simulink model "RailP_DD"  (R2018a)
settings: configuration reference "cs_ert" (kept outside this file)
model workspace (MAT data in the model file):
  RailP_DD_DT = 10
values from neighbouring files (symbols this model uses):
  RailP_pLin_CUR : value not decoded    [RailP_DD.sldd]
  RailP_pLin_CURX : value not decoded    [RailP_DD.sldd]
  RailP_tiSRCMaxDefDeb_C = 200.0    [RailP_DD.sldd]
  RailP_tiSRCMaxOKDeb_C = 200.0    [RailP_DD.sldd]
  RailP_tiSRCMinDefDeb_C = 200.0    [RailP_DD.sldd]
  RailP_tiSRCMinOKDeb_C = 200.0    [RailP_DD.sldd]
  RailP_uSRCMax_C = 4700.0    [RailP_DD.sldd]
  RailP_uSRCMin_C = 131.0    [RailP_DD.sldd]
libraries: sllib x2
settings Model: DataDictionary=RailP_DD.sldd  Creator=zhoutinglin  LastModifiedBy=zhoutinglin

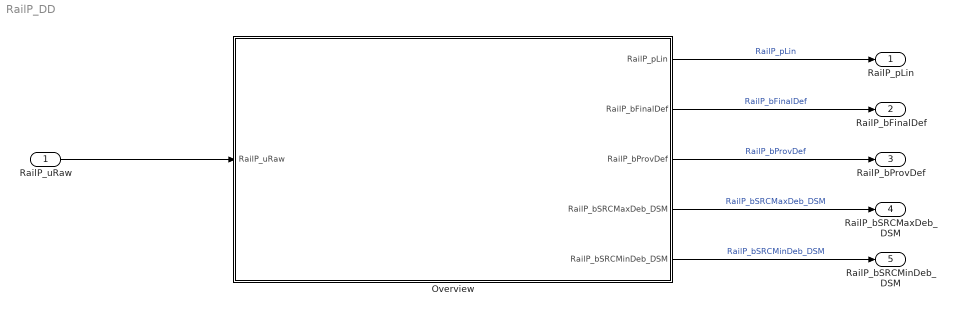
== system RailP_DD ==
  RailP_uRaw : Inport  Description=Status of FId_RailPSS  OutMin=0  OutMax=5000  OutDataTypeStr=Volt_mV  PortDimensions=[1 1]
  Overview : Subsystem
  RailP_pLin : Outport
  RailP_bFinalDef : Outport  Port=2
  RailP_bProvDef : Outport  Port=3
  RailP_bSRCMaxDeb_DSM : Outport  Port=4
  RailP_bSRCMinDeb_DSM : Outport  Port=5
  wires:
  RailP_uRaw/1 -> Overview/1(RailP_uRaw)
  Overview/1(RailP_pLin) -> RailP_pLin/1  "RailP_pLin"
  Overview/2(RailP_bFinalDef) -> RailP_bFinalDef/1  "RailP_bFinalDef"
  Overview/3(RailP_bProvDef) -> RailP_bProvDef/1  "RailP_bProvDef"
  Overview/4(RailP_bSRCMaxDeb_DSM) -> RailP_bSRCMaxDeb_DSM/1  "RailP_bSRCMaxDeb_DSM"
  Overview/5(RailP_bSRCMinDeb_DSM) -> RailP_bSRCMinDeb_DSM/1  "RailP_bSRCMinDeb_DSM"

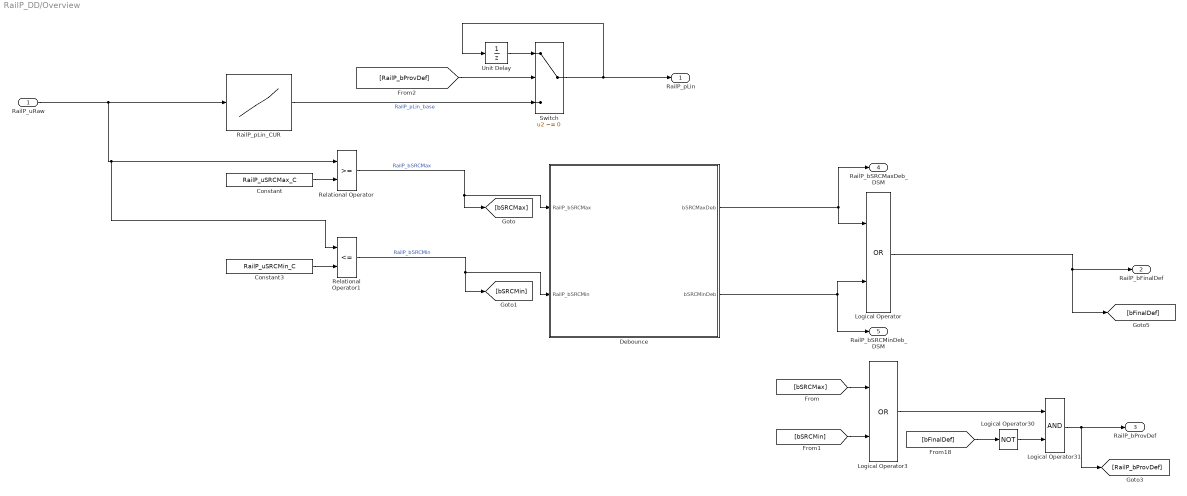
== system RailP_DD/Overview ==
  RailP_uRaw : Inport  Tag=mv
  Constant : Constant  Value=RailP_uSRCMax_C
  Constant3 : Constant  Value=RailP_uSRCMin_C
  Debounce : Subsystem
  Logical Operator : Logic  Operator=OR  AllPortsSameDT=off  OutDataTypeStr=boolean
  Logical Operator3 : Logic  Operator=OR  AllPortsSameDT=off  OutDataTypeStr=boolean
  Logical Operator30 : Logic  Operator=NOT  AllPortsSameDT=off  OutDataTypeStr=boolean
  Logical Operator31 : Logic  AllPortsSameDT=off  OutDataTypeStr=boolean
  RailP_pLin_CUR : Lookup_n-D  NumberOfTableDimensions=1  BreakpointsForDimension1=RailP_pLin_CURX  IndexSearchMethod=Linear search  BeginIndexSearchUsingPreviousIndexResult=on  UseOneInputPortForAllInputData=on  Table=RailP_pLin_CUR  ExtrapMethod=Clip  UseLastTableValue=on  InternalRulePriority=Speed  OutDataTypeStr=Inherit: Inherit via back propagation  SaturateOnIntegerOverflow=on
  Relational Operator : RelationalOperator  OutDataTypeStr=boolean  RndMeth=Nearest  InputSameDT=on
  Relational Operator1 : RelationalOperator  Operator=<=  OutDataTypeStr=boolean  RndMeth=Nearest  InputSameDT=on
  Switch : Switch  Criteria=u2 ~= 0
  Unit Delay : UnitDelay  SampleTime=-1
      settings: AttributesFormatString=InitialValue=%<InitialCondition>
  RailP_pLin : Outport  Tag=bar
  RailP_bFinalDef : Outport  Port=2
  RailP_bProvDef : Outport  Port=3
  RailP_bSRCMaxDeb_DSM : Outport  Port=4
  RailP_bSRCMinDeb_DSM : Outport  Port=5
  wires:
  Relational Operator1/1 -> [bSRCMin], Debounce/2(RailP_bSRCMin)  "RailP_bSRCMin"
  RailP_pLin_CUR/1 -> Switch/3  "RailP_pLin_base"
  [RailP_bProvDef] -> Switch/2
  Constant/1 -> Relational Operator/2
  Debounce/2(bSRCMinDeb) -> Logical Operator/2, RailP_bSRCMinDeb_DSM/1
  Switch/1 -> Unit Delay/1, RailP_pLin/1
  Logical Operator/1 -> [bFinalDef], RailP_bFinalDef/1
  Debounce/1(bSRCMaxDeb) -> Logical Operator/1, RailP_bSRCMaxDeb_DSM/1
  [bSRCMin] -> Logical Operator3/2
  Unit Delay/1 -> Switch/1
  [bSRCMax] -> Logical Operator3/1
  [bFinalDef] -> Logical Operator30/1
  Logical Operator3/1 -> Logical Operator31/1
  Logical Operator30/1 -> Logical Operator31/2
  Relational Operator/1 -> [bSRCMax], Debounce/1(RailP_bSRCMax)  "RailP_bSRCMax"
  Logical Operator31/1 -> [RailP_bProvDef], RailP_bProvDef/1
  RailP_uRaw/1 -> Relational Operator1/1, Relational Operator/1, RailP_pLin_CUR/1
  Constant3/1 -> Relational Operator1/2

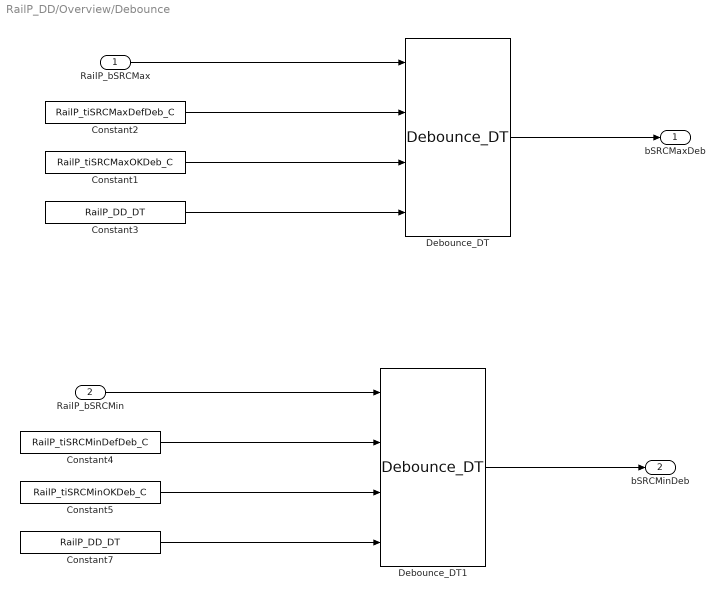
== system RailP_DD/Overview/Debounce ==
  RailP_bSRCMax : Inport
  RailP_bSRCMin : Inport  Port=2
  Constant1 : Constant  Value=RailP_tiSRCMaxOKDeb_C
  Constant2 : Constant  Value=RailP_tiSRCMaxDefDeb_C
  Constant3 : Constant  Value=RailP_DD_DT  OutDataTypeStr=Inherit: Inherit via back propagation
  Constant4 : Constant  Value=RailP_tiSRCMinDefDeb_C
  Constant5 : Constant  Value=RailP_tiSRCMinOKDeb_C
  Constant7 : Constant  Value=RailP_DD_DT  OutDataTypeStr=Inherit: Inherit via back propagation
  Debounce_DT : sllib/Debounce_DT
      settings: SourceProductName=sllib
  Debounce_DT1 : sllib/Debounce_DT
      settings: SourceProductName=sllib
  bSRCMaxDeb : Outport
  bSRCMinDeb : Outport  Port=2
  wires:
  Constant7/1 -> Debounce_DT1/4
  Constant3/1 -> Debounce_DT/4
  RailP_bSRCMax/1 -> Debounce_DT/1
  Constant5/1 -> Debounce_DT1/3
  RailP_bSRCMin/1 -> Debounce_DT1/1
  Constant1/1 -> Debounce_DT/3
  Constant4/1 -> Debounce_DT1/2
  Debounce_DT/1 -> bSRCMaxDeb/1
  Debounce_DT1/1 -> bSRCMinDeb/1
  Constant2/1 -> Debounce_DT/2
